simulink model "rct_airframeTRIM"  (R2016b)
settings: Solver=ode45  StartTime=0.0  StopTime=1  RelTol=1e-3  AbsTol=1e-6
model workspace (MATLAB code in the model file):
  | AirframeData
  | x_ini = 0;                          % Initial downrange position [m]
  | h_ini = 10000/3.28084;    % Trim Height=10,000ft [m]
  | theta_ini  = 0;                   % Initial pitch angle [rad]
  | q_ini = 0;                           % Initial pitch rate [rad/sec]
undefined symbols (not defined in the file or in its folder): Cm_alpha, Cm_el, Cm_q, Cx_alpha, Cz_alpha, Cz_el, d_ref, g, S_ref, Thrust
libraries: aerospace x3
settings Model: ExtModeTrigMode=oneshot  ExtModeArmWhenConnect=off  ExtModeAutoUpdateStatusClock=off  Creator=The MathWorks, Inc.  LastModifiedBy=The MathWorks, Inc.
settings DataIOCC: SaveFormat=Array  SignalLoggingName=sigsOut
settings OptimizationCC: BlockReduction=off  BooleanDataType=off  ExpressionDepthLimit=2147483647  InitFltsAndDblsToZero=on  LifeSpan=inf
settings DebuggingCC: SaveWithParameterizedLinksMsg=none  UnderspecifiedInitializationDetection=Classic  MergeDetectMultiDrivingBlocksExec=none  CheckExecutionContextPreStartOutputMsg=on  CheckExecutionContextRuntimeOutputMsg=on  SignalResolutionControl=TryResolveAllWithWarning  MultiTaskDSMMsg=warning  FcnCallInpInsideContextMsg=warning  AllowSymbolicDim=off  StateNameClashWarn=warning  StrictBusMsg=None  SFUnexpectedBacktrackingDiag=warning  SFNoUnconditionalDefaultTransitionDiag=warning  SFExecutionAtInitializationDiag=none
settings HardwareCC: ProdBitPerPointer=32  ProdBitPerSizeT=32  ProdBitPerPtrDiffT=32  ProdLargestAtomicFloat=None  ProdIntDivRoundTo=Undefined  ProdEndianess=Unspecified  ProdWordSize=32  ProdHWDeviceType=32-bit Generic  TargetUnknown=on
settings ModelReferenceCC: PropagateSignalLabelsOutOfModel=off
settings GRTTargetCC: TargetFcnLib=ansi_tfl_tmw.mat  TargetLangStandard=C89/C90 (ANSI)  GeneratePreprocessorConditionals=Disable all  CombineOutputUpdateFcns=off  GRTInterface=on
settings ConfigComp: CovMetricSettings=dw  CovHtmlReporting=on  CovSaveCumulativeToWorkspaceVar=on  CovSaveSingleToWorkspaceVar=on  CovExternalEMLEnable=off

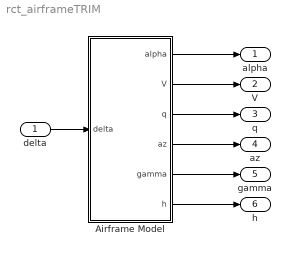
== system rct_airframeTRIM ==
  delta : Inport
  Airframe Model : Subsystem
  alpha : Outport  InitialOutput=0
  V : Outport  Port=2  InitialOutput=0
  q : Outport  Port=3  InitialOutput=0
  az : Outport  Port=4  InitialOutput=0
  gamma : Outport  Port=5  InitialOutput=0
  h : Outport  Port=6  InitialOutput=0
  wires:
  delta/1 -> Airframe Model/1(delta)
  Airframe Model/4(az) -> az/1
  Airframe Model/3(q) -> q/1
  Airframe Model/5(gamma) -> gamma/1
  Airframe Model/1(alpha) -> alpha/1
  Airframe Model/2(V) -> V/1
  Airframe Model/6(h) -> h/1

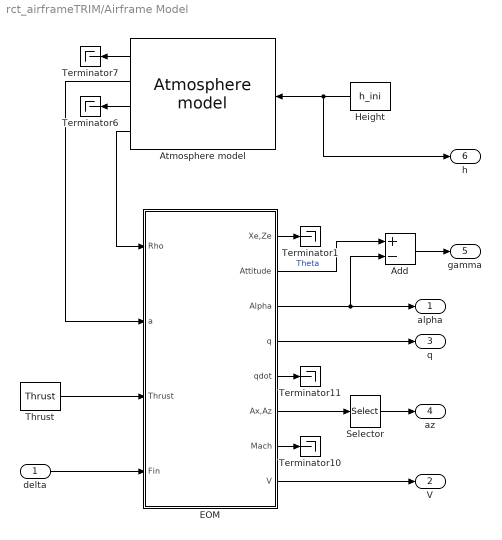
== system rct_airframeTRIM/Airframe Model ==
  delta : Inport
  Add : Sum  Inputs=+-
  Atmosphere model : aerospace/Atmosphere/Atmosphere model
  EOM : Subsystem
  Height : Constant  Value=h_ini
  Selector : Selector  InputPortWidth=2  IndexOptions=Index vector (dialog)  Indices=[2]  OutputSizes=1
  Terminator{1,6..7,10..11} (5 alike) : Terminator
  Thrust : Constant  Value=Thrust
  alpha : Outport  InitialOutput=0
  V : Outport  Port=2  InitialOutput=0
  q : Outport  Port=3  InitialOutput=0
  az : Outport  Port=4  InitialOutput=0
  gamma : Outport  Port=5  InitialOutput=0
  h : Outport  Port=6
  wires:
  Add/1 -> gamma/1
  EOM/2(Attitude) -> Add/1  "Theta"
  EOM/6(Ax,Az) -> Selector/1
  EOM/3(Alpha) -> Add/2, alpha/1
  Thrust/1 -> EOM/3(Thrust)
  EOM/1(Xe,Ze) -> Terminator1/1
  EOM/4(q) -> q/1
  EOM/5(qdot) -> Terminator11/1
  EOM/7(Mach) -> Terminator10/1
  Atmosphere model/4 -> EOM/1(Rho)
  Atmosphere model/2 -> EOM/2(a)
  Selector/1 -> az/1
  EOM/8(V) -> V/1
  delta/1 -> EOM/4(Fin)
  Atmosphere model/3 -> Terminator6/1
  Atmosphere model/1 -> Terminator7/1
  Height/1 -> h/1, Atmosphere model/1

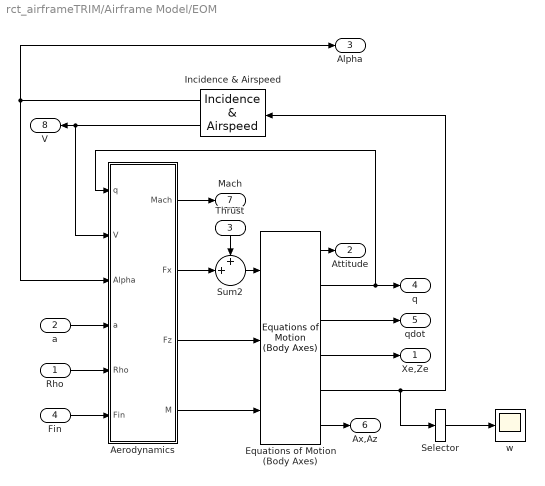
== system rct_airframeTRIM/Airframe Model/EOM ==
  Rho : Inport
  a : Inport  Port=2
  Thrust : Inport  Port=3
  Fin : Inport  Port=4
  " Equations of Motion (Body Axes)" : aerospace/3DoF Equations of Motion / Equations of Motion (Body Axes)  v_ini=v_ini  theta_ini=theta_ini  alpha_ini=alpha_ini  q_ini=q_ini  pos_ini=[x_ini -h_ini]  mass=mass  Iyy=Iyy  g=g
  Aerodynamics : Subsystem
  Incidence & Airspeed : aerospace/3DoF Equations of Motion /Incidence  & Airspeed
  Selector : Selector  InputPortWidth=2  IndexOptions=Index vector (dialog)  Indices=[2]  OutputSizes=1
  Sum2 : Sum  Inputs=++|  SaturateOnIntegerOverflow=on  InputSameDT=on  OutDataTypeStr=Inherit: Same as first input
  w : Scope
  Xe,Ze : Outport  InitialOutput=0
  Attitude : Outport  Port=2  InitialOutput=0
  Alpha : Outport  Port=3  InitialOutput=0
  q : Outport  Port=4  InitialOutput=0
  qdot : Outport  Port=5  InitialOutput=0
  Ax,Az : Outport  Port=6  InitialOutput=0
  Mach : Outport  Port=7  InitialOutput=0
  V : Outport  Port=8  InitialOutput=0
  wires:
  Selector/1 -> w/1
  Aerodynamics/1(" Mach") -> Mach/1
  Aerodynamics/4(" M") -> " Equations of Motion (Body Axes)"/3
  Sum2/1 -> " Equations of Motion (Body Axes)"/1
  Incidence & Airspeed/1 -> Aerodynamics/3(Alpha), Alpha/1
  Rho/1 -> Aerodynamics/5(Rho)
  a/1 -> Aerodynamics/4(a)
  Fin/1 -> Aerodynamics/6(Fin)
  Incidence & Airspeed/2 -> V/1, Aerodynamics/2(V)
  Aerodynamics/3(Fz) -> " Equations of Motion (Body Axes)"/2
  Aerodynamics/2(Fx) -> Sum2/2
  Thrust/1 -> Sum2/1
  " Equations of Motion (Body Axes)"/2 -> q/1, Aerodynamics/1(q)
  " Equations of Motion (Body Axes)"/3 -> qdot/1
  " Equations of Motion (Body Axes)"/1 -> Attitude/1
  " Equations of Motion (Body Axes)"/4 -> Xe,Ze/1
  " Equations of Motion (Body Axes)"/6 -> Ax,Az/1
  " Equations of Motion (Body Axes)"/5 -> Incidence & Airspeed/1, Selector/1

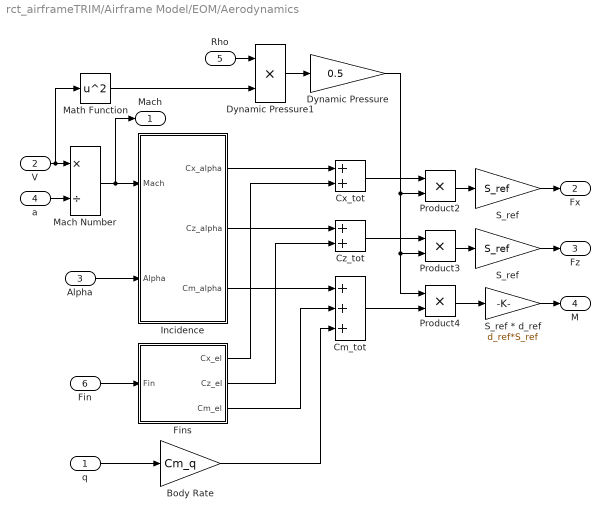
== system rct_airframeTRIM/Airframe Model/EOM/Aerodynamics ==
  q : Inport
  V : Inport  Port=2
  Alpha : Inport  Port=3
  a : Inport  Port=4
  Rho : Inport  Port=5
  Fin : Inport  Port=6
  Body Rate : Gain  Gain=Cm_q  SaturateOnIntegerOverflow=on  OutDataTypeStr=Inherit: Same as input  ParamDataTypeStr=Inherit: Same as input
  Cm_tot : Sum  Inputs=+++  SaturateOnIntegerOverflow=on  InputSameDT=on  OutDataTypeStr=Inherit: Same as first input
  Cx_tot : Sum  SaturateOnIntegerOverflow=on  InputSameDT=on  OutDataTypeStr=Inherit: Same as first input
  Cz_tot : Sum  SaturateOnIntegerOverflow=on  InputSameDT=on  OutDataTypeStr=Inherit: Same as first input
  Dynamic Pressure : Gain  Gain=0.5  SaturateOnIntegerOverflow=on  OutDataTypeStr=Inherit: Same as input  ParamDataTypeStr=Inherit: Same as input
  Dynamic Pressure1 : Product  SaturateOnIntegerOverflow=on  InputSameDT=on  OutDataTypeStr=Inherit: Same as first input
  Fins : Subsystem
  Incidence : Subsystem
  Mach Number : Product  Inputs=*/  SaturateOnIntegerOverflow=on  InputSameDT=on  OutDataTypeStr=Inherit: Same as first input
  Math Function : Math  Operator=square  SaturateOnIntegerOverflow=on
  Product2 : Product  SaturateOnIntegerOverflow=on  InputSameDT=on  OutDataTypeStr=Inherit: Same as first input
  Product3 : Product  SaturateOnIntegerOverflow=on  InputSameDT=on  OutDataTypeStr=Inherit: Same as first input
  Product4 : Product  SaturateOnIntegerOverflow=on  InputSameDT=on  OutDataTypeStr=Inherit: Same as first input
  S_ref : Gain  Gain=S_ref  SaturateOnIntegerOverflow=on  OutDataTypeStr=Inherit: Same as input  ParamDataTypeStr=Inherit: Same as input
  S_ref * d_ref : Gain  Gain=d_ref*S_ref  SaturateOnIntegerOverflow=on  OutDataTypeStr=Inherit: Same as input  ParamDataTypeStr=Inherit: Same as input
  "S_ref " : Gain  Gain=S_ref  SaturateOnIntegerOverflow=on  OutDataTypeStr=Inherit: Same as input  ParamDataTypeStr=Inherit: Same as input
  " Mach" : Outport  InitialOutput=0
  Fx : Outport  Port=2  InitialOutput=[0]
  Fz : Outport  Port=3  InitialOutput=0
  " M" : Outport  Port=4  InitialOutput=0
  wires:
  Math Function/1 -> Dynamic Pressure1/2
  Rho/1 -> Dynamic Pressure1/1
  Dynamic Pressure1/1 -> Dynamic Pressure/1
  Dynamic Pressure/1 -> Product2/2, Product3/2, Product4/1
  V/1 -> Math Function/1, Mach Number/1
  Incidence/1(Cx_alpha) -> Cx_tot/1
  Fins/1(Cx_el) -> Cx_tot/2
  Incidence/2(Cz_alpha) -> Cz_tot/1
  Fins/2(Cz_el) -> Cz_tot/2
  Incidence/3(Cm_alpha) -> Cm_tot/1
  Fins/3(Cm_el) -> Cm_tot/2
  Body Rate/1 -> Cm_tot/3
  a/1 -> Mach Number/2
  Alpha/1 -> Incidence/2(Alpha)
  Cx_tot/1 -> Product2/1
  Cz_tot/1 -> Product3/1
  Product2/1 -> S_ref/1
  S_ref/1 -> Fx/1
  Product3/1 -> "S_ref "/1
  "S_ref "/1 -> Fz/1
  Fin/1 -> Fins/1(Fin)
  S_ref * d_ref/1 -> " M"/1
  Product4/1 -> S_ref * d_ref/1
  Cm_tot/1 -> Product4/2
  q/1 -> Body Rate/1
  Mach Number/1 -> " Mach"/1, Incidence/1(Mach)

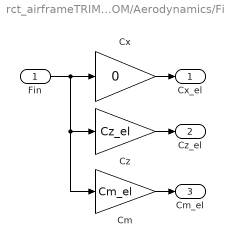
== system rct_airframeTRIM/Airframe Model/EOM/Aerodynamics/Fins ==
  Fin : Inport
  Cm : Gain  Gain=Cm_el  SaturateOnIntegerOverflow=on  OutDataTypeStr=Inherit: Same as input  ParamDataTypeStr=Inherit: Same as input
  Cx : Gain  Gain=0  SaturateOnIntegerOverflow=on  OutDataTypeStr=Inherit: Same as input  ParamDataTypeStr=Inherit: Same as input
  Cz : Gain  Gain=Cz_el  SaturateOnIntegerOverflow=on  OutDataTypeStr=Inherit: Same as input  ParamDataTypeStr=Inherit: Same as input
  Cx_el : Outport  InitialOutput=0
  Cz_el : Outport  Port=2  InitialOutput=0
  Cm_el : Outport  Port=3  InitialOutput=0
  wires:
  Fin/1 -> Cx/1, Cm/1, Cz/1
  Cx/1 -> Cx_el/1
  Cm/1 -> Cm_el/1
  Cz/1 -> Cz_el/1

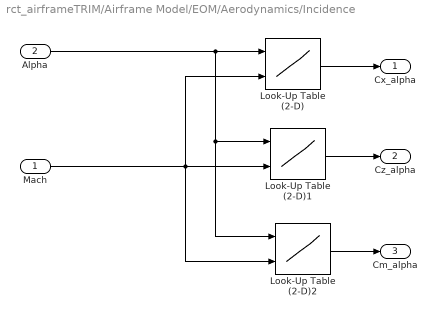
== system rct_airframeTRIM/Airframe Model/EOM/Aerodynamics/Incidence ==
  Mach : Inport
  Alpha : Inport  Port=2
  Look-Up Table (2-D) : Lookup2D  RowIndex=alpha_vec  ColumnIndex=Mach_vec  Table=Cx_alpha  SaturateOnIntegerOverflow=on
  Look-Up Table (2-D)1 : Lookup2D  RowIndex=alpha_vec  ColumnIndex=Mach_vec  Table=Cz_alpha  SaturateOnIntegerOverflow=on
  Look-Up Table (2-D)2 : Lookup2D  RowIndex=alpha_vec  ColumnIndex=Mach_vec  Table=Cm_alpha  SaturateOnIntegerOverflow=on
  Cx_alpha : Outport  InitialOutput=0
  Cz_alpha : Outport  Port=2  InitialOutput=0
  Cm_alpha : Outport  Port=3  InitialOutput=0
  wires:
  Look-Up Table (2-D)/1 -> Cx_alpha/1
  Look-Up Table (2-D)1/1 -> Cz_alpha/1
  Look-Up Table (2-D)2/1 -> Cm_alpha/1
  Alpha/1 -> Look-Up Table (2-D)/1, Look-Up Table (2-D)1/1, Look-Up Table (2-D)2/1
  Mach/1 -> Look-Up Table (2-D)/2, Look-Up Table (2-D)1/2, Look-Up Table (2-D)2/2
